simulink model "ex3_sim1"  (R2022b)
settings: Solver=ode45  StartTime=0.0  StopTime=3  MaxStep=0.0001  RelTol=1e-3
undefined symbols (not defined in the file): denCd, denP, DiscIntNeverNeededParam, numCd, numP, pid, sig, Ts, umax
settings Model: Creator=Lorenzo  LastModifiedBy=loren
settings DataIOCC: ReturnWorkspaceOutputs=off

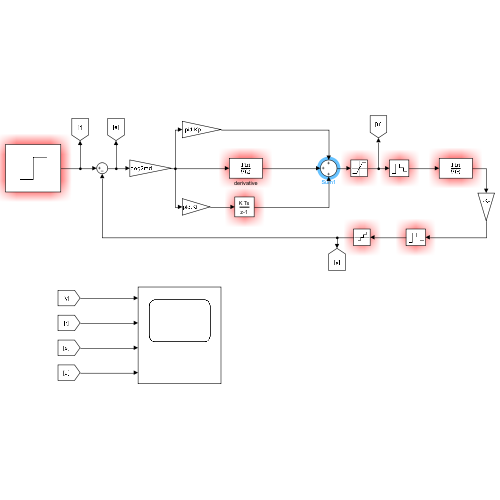
[thumbnail: Simulink's stored preview of the top-level diagram]
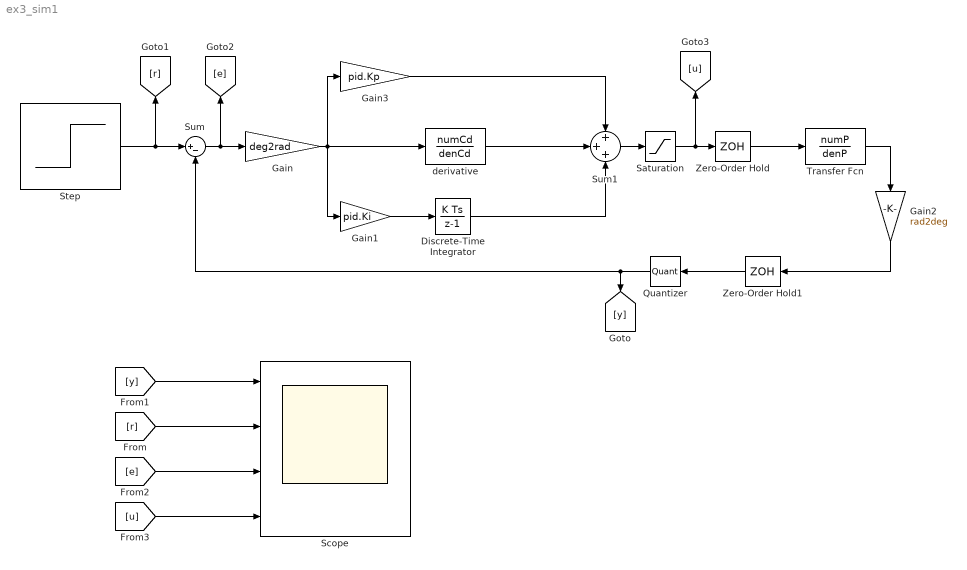
== system ex3_sim1 ==
  Discrete-Time Integrator : DiscreteIntegrator  SampleTime=Ts  ICPrevOutput=DiscIntNeverNeededParam  ICPrevScaledInput=DiscIntNeverNeededParam
  Gain : Gain  Gain=deg2rad
  Gain1 : Gain  Gain=pid.Ki
  Gain2 : Gain  Gain=rad2deg
  Gain3 : Gain  Gain=pid.Kp
  Quantizer : Quantizer  QuantizationInterval=pulse2deg
  Saturation : Saturate  UpperLimit=umax  LowerLimit=-umax
  Scope : Scope  NumInputPorts=4
  Step : Step  Time=sig.t  After=sig.A  SampleTime=0
  Sum : Sum  Inputs=|+-
  Sum1 : Sum  Inputs=+++
  Transfer Fcn : TransferFcn  Numerator=numP  Denominator=denP
  Zero-Order Hold : ZeroOrderHold  SampleTime=Ts
  Zero-Order Hold1 : ZeroOrderHold  SampleTime=Ts
  derivative : DiscreteTransferFcn  Numerator=numCd  Denominator=denCd  SampleTime=Ts
  wires:
  Step/1 -> [r], Sum/1
  Sum/1 -> [e], Gain/1
  Zero-Order Hold/1 -> Transfer Fcn/1
  Transfer Fcn/1 -> Gain2/1
  Zero-Order Hold1/1 -> Quantizer/1
  Saturation/1 -> [u], Zero-Order Hold/1
  Sum1/1 -> Saturation/1
  Gain/1 -> derivative/1, Gain3/1, Gain1/1
  Quantizer/1 -> Sum/2, [y]
  [r] -> Scope/2
  [y] -> Scope/1
  [e] -> Scope/3
  [u] -> Scope/4
  derivative/1 -> Sum1/2
  Gain3/1 -> Sum1/1
  Discrete-Time Integrator/1 -> Sum1/3
  Gain1/1 -> Discrete-Time Integrator/1
  Gain2/1 -> Zero-Order Hold1/1
